simulink model "cell_model_nmc"  (R2024b)
settings: Solver=FixedStepDiscrete  StartTime=0.0  StopTime=600  FixedStep=1  RelTol=1e-3
settings Model: Creator=rayen  LastModifiedBy=rayen

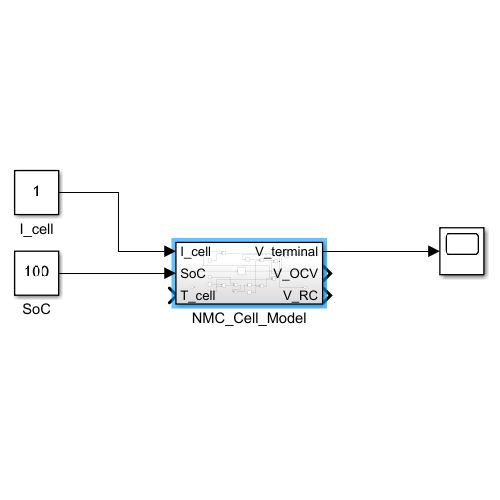
[thumbnail: Simulink's stored preview of the top-level diagram]
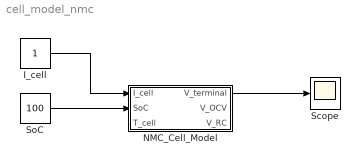
== system cell_model_nmc ==
  I_cell : Constant
  NMC_Cell_Model : Subsystem
  Scope : Scope
  SoC : Constant  Value=100
  wires:
  SoC/1 -> NMC_Cell_Model/2(SoC)
  I_cell/1 -> NMC_Cell_Model/1(I_cell)
  NMC_Cell_Model/1(V_terminal) -> Scope/1

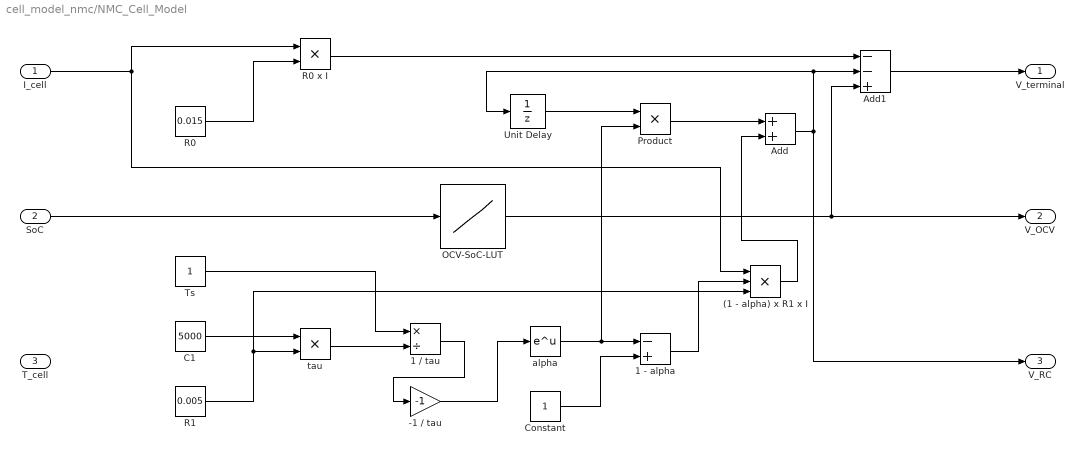
== system cell_model_nmc/NMC_Cell_Model ==
  I_cell : Inport
  SoC : Inport  Port=2
  T_cell : Inport  Port=3
  (1 - alpha) x R1 x I : Product  Inputs=3
  -1 / tau : Gain  Gain=-1
  1 - alpha : Sum  Inputs=-+
  1 / tau : Product  Inputs=*/
  Add : Sum
  Add1 : Sum  Inputs=--+
  C1 : Constant  Value=5000
  Constant : Constant
  OCV-SoC-LUT : Lookup_n-D  NumberOfTableDimensions=1  BreakpointsForDimension1=[0, 5, 10, 20, 30, 40, 50, 60, 70, 80, 90, 95, 100]  Table=[2.50, 3.30, 3.45, 3.55, 3.60, 3.63, 3.65, 3.70, 3.78, 3.90, 4.05, 4.15, 4.20]  ExtrapMethod=Clip  InternalRulePriority=Speed  RndMeth=Simplest
  Product : Product
  R0 : Constant  Value=0.015
  R0 x I : Product
  R1 : Constant  Value=0.005
  Ts : Constant
  Unit Delay : UnitDelay  HasFrameUpgradeWarning=on
  alpha : Math
  tau : Product
  V_terminal : Outport
  V_OCV : Outport  Port=2
  V_RC : Outport  Port=3
  wires:
  SoC/1 -> OCV-SoC-LUT/1
  OCV-SoC-LUT/1 -> Add1/3, V_OCV/1
  I_cell/1 -> (1 - alpha) x R1 x I/1, R0 x I/1
  R0/1 -> R0 x I/2
  C1/1 -> tau/1
  R1/1 -> tau/2, (1 - alpha) x R1 x I/3
  tau/1 -> 1 / tau/2
  Ts/1 -> 1 / tau/1
  1 / tau/1 -> -1 / tau/1
  -1 / tau/1 -> alpha/1
  alpha/1 -> Product/2, 1 - alpha/1
  Constant/1 -> 1 - alpha/2
  1 - alpha/1 -> (1 - alpha) x R1 x I/2
  (1 - alpha) x R1 x I/1 -> Add/2
  R0 x I/1 -> Add1/1
  Unit Delay/1 -> Product/1
  Product/1 -> Add/1
  Add/1 -> V_RC/1, Add1/2, Unit Delay/1
  Add1/1 -> V_terminal/1
